simulink model "draftS_base"  (R2023b)
settings: Solver=ode4  StartTime=0.0  StopTime=0.5  FixedStep=Ts  RelTol=1e-3
undefined symbols (not defined in the file): Ts
libraries: spsMeanLib x7, spsCurrentMeasurementLib x4, spsVoltageMeasurementLib x3, spsSeriesRLCBranchLib x3, spsDCVoltageSourceLib x1, spsDiodeLib x1, spsGroundLib x1, spsMosfetLib x1, spsPWMGeneratorDCDCLib x1, sps_lib x1
settings Model: Creator=ssbor  LastModifiedBy=ssbor

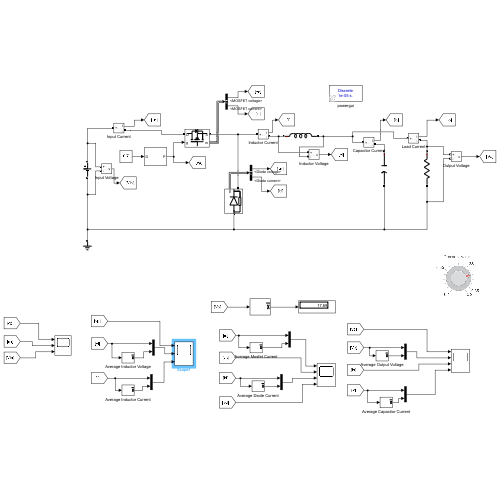
[thumbnail: Simulink's stored preview of the top-level diagram]
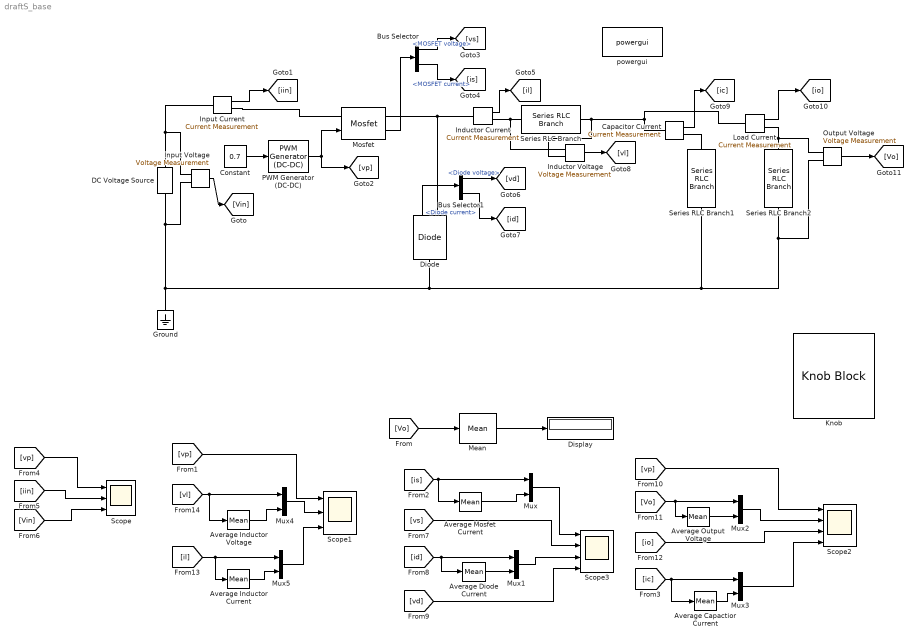
== system draftS_base ==
  Average Capactior Current : spsMeanLib/Mean  Freq=15000  Vinit=0  Ts=0
  Average Diode Current : spsMeanLib/Mean  Freq=15000  Vinit=0  Ts=0
  Average Inductor Current : spsMeanLib/Mean  Freq=15000  Vinit=0  Ts=0
  Average Inductor Voltage : spsMeanLib/Mean  Freq=15000  Vinit=0  Ts=0
      link override Model/Transport Delay: DelayTime=1./sps.Freq
  Average Mosfet Current : spsMeanLib/Mean  Freq=15000  Vinit=0  Ts=0
  Average Output Voltage : spsMeanLib/Mean  Freq=15000  Vinit=0  Ts=0
  Bus Selector : BusSelector  OutputSignals=MOSFET voltage,MOSFET current
  Bus Selector1 : BusSelector  OutputSignals=Diode voltage,Diode current
  Capacitor Current : spsCurrentMeasurementLib/Current Measurement  PhasorSimulation=off  OutputType=Complex  PSBequivalent=0
  Constant : Constant  Value=0.7
  DC Voltage Source : spsDCVoltageSourceLib/DC Voltage Source  Amplitude=25  Measurements=None
  Diode : spsDiodeLib/Diode  Ron=1e-7  Lon=0  Vf=0  IC=0  UseSnubber=0  Rs=1e6  Cs=1e6  Measurements=on
  Display : Display
  Ground : spsGroundLib/Ground  LConnTagsString=a
  Inductor Current : spsCurrentMeasurementLib/Current Measurement  PhasorSimulation=off  OutputType=Complex  PSBequivalent=0
  Inductor Voltage : spsVoltageMeasurementLib/Voltage Measurement  PhasorSimulation=off  OutputType=Complex  PSBequivalent=0
  Input Current : spsCurrentMeasurementLib/Current Measurement  PhasorSimulation=off  OutputType=Complex  PSBequivalent=0
  Input Voltage : spsVoltageMeasurementLib/Voltage Measurement  PhasorSimulation=off  OutputType=Complex  PSBequivalent=0
  Knob : KnobBlock  ScaleMin=0.1  ScaleMax=0.9  TickInterval=0.25
  Load Current : spsCurrentMeasurementLib/Current Measurement  PhasorSimulation=off  OutputType=Complex  PSBequivalent=0
  Mean : spsMeanLib/Mean  Freq=15000  Vinit=0  Ts=0
  Mosfet : spsMosfetLib/Mosfet  Ron=1e-7  Lon=0  Rd=1e-10  Vfd=0  IC=0  Rs=inf  Cs=0  Measurements=on
  Mux{,1..5} (6 alike) : Mux  Inputs=2
  Output Voltage : spsVoltageMeasurementLib/Voltage Measurement  PhasorSimulation=off  OutputType=Complex  PSBequivalent=0
  PWM Generator (DC-DC) : spsPWMGeneratorDCDCLib/PWM Generator (DC-DC)  Fsw=15000  Ts=Ts
  Scope : Scope  NumInputPorts=3
  Scope1 : Scope  NumInputPorts=3
  Scope2 : Scope  NumInputPorts=4
  Scope3 : Scope  NumInputPorts=4
  Series RLC Branch : spsSeriesRLCBranchLib/Series RLC Branch  LConnTagsString=__new0  RConnTagsString=__new0  BranchType=L  Resistance=1  Inductance=0.001  SetiL0=off  InitialCurrent=0  Capacitance=1e-6  Setx0=off  InitialVoltage=0  Measurements=None
  Series RLC Branch1 : spsSeriesRLCBranchLib/Series RLC Branch  LConnTagsString=__new0  RConnTagsString=__new0  BranchType=C  Resistance=1  Inductance=1e-3  SetiL0=off  InitialCurrent=0  Capacitance=470e-6  Setx0=off  InitialVoltage=0  Measurements=None
  Series RLC Branch2 : spsSeriesRLCBranchLib/Series RLC Branch  LConnTagsString=__new0  RConnTagsString=__new0  BranchType=R  Resistance=20  Inductance=1e-3  SetiL0=off  InitialCurrent=0  Capacitance=1e-6  Setx0=off  InitialVoltage=0  Measurements=None
  powergui : sps_lib/powergui  Priority=1  SimulationMode=Discrete  SampleTime=Ts  frequency=60  Iterations=50  frequencyindice=0  Pbase=100e6  ErrMax=1e-4  UnitsV=kV  UnitsW=MW  buscounter=0  FunctionMessages=off  echomessages=off  EnableUseOfTLC=off  CurrentSourceSwitches=off  DisableSnubberDevices=off  DisableRonSwitches=off  DisableVfSwitches=off  DisplayEquations=off  AutomaticDiscreteSolvers=off  SolverType=Tustin/Backward Euler (TBE)  Interpol=off  ExternalGateDelay=off  methode=off  Ts=100  x0status=blocks  SPID=on  SwTol=0  HookPort=off  NonlinearTolerance=1e-4  nMaxIteration=100  ContinueOnMaxIteration=off  RestoreLinks=warning  ResistiveCurrentMeasurement=off  Frange=[0:2:500]  Ylog=off  Xlog=on  ShowGrid=off  save=off  variable=ZData  structure=0  ZoomFFT=off  StartTime=0.0  cycles=1  DisplayStyle=1  fundamental=60  FreqAxis=off  MaxFrequency=1000  frequencyindicesteady=1  RmsSteady=1  display=off
  wires:
  Input Voltage/1 -> [Vin]
  Input Current/1 -> [iin]
  Constant/1 -> PWM Generator (DC-DC)/1
  PWM Generator (DC-DC)/1 -> [vp], Mosfet/1
  Mosfet/1 -> Bus Selector/1
  Bus Selector/1 -> [vs]  "<MOSFET voltage>"
  Bus Selector/2 -> [is]  "<MOSFET current>"
  Inductor Current/1 -> [il]
  Capacitor Current/1 -> [ic]
  Inductor Voltage/1 -> [vl]
  Load Current/1 -> [io]
  Output Voltage/1 -> [Vo]
  Diode/1 -> Bus Selector1/1
  Bus Selector1/1 -> [vd]  "<Diode voltage>"
  Bus Selector1/2 -> [id]  "<Diode current>"
  [Vo] -> Mean/1
  Mean/1 -> Display/1
  [vp] -> Scope/1
  [iin] -> Scope/2
  [Vin] -> Scope/3
  [vs] -> Scope3/2
  [vd] -> Scope3/4
  [vp] -> Scope2/1
  [io] -> Scope2/3
  Average Mosfet Current/1 -> Mux/2
  [is] -> Mux/1, Average Mosfet Current/1
  Mux/1 -> Scope3/1
  [id] -> Average Diode Current/1, Mux1/1
  Average Diode Current/1 -> Mux1/2
  Mux1/1 -> Scope3/3
  [Vo] -> Average Output Voltage/1, Mux2/1
  Average Output Voltage/1 -> Mux2/2
  Mux2/1 -> Scope2/2
  [ic] -> Average Capactior Current/1, Mux3/1
  Average Capactior Current/1 -> Mux3/2
  Mux3/1 -> Scope2/4
  [vp] -> Scope1/1
  [vl] -> Average Inductor Voltage/1, Mux4/1
  Average Inductor Voltage/1 -> Mux4/2
  Mux4/1 -> Scope1/2
  [il] -> Mux5/1, Average Inductor Current/1
  Average Inductor Current/1 -> Mux5/2
  Mux5/1 -> Scope1/3
  connections:
  DC Voltage Source/RConn1 -- Input Voltage/LConn1 -- Input Current/LConn1
  DC Voltage Source/LConn1 -- Input Voltage/LConn2 -- Ground/LConn1 -- Series RLC Branch2/RConn1 -- Output Voltage/LConn2 -- Series RLC Branch1/RConn1 -- Diode/LConn1
  Input Current/RConn1 -- Mosfet/LConn1
  Mosfet/RConn1 -- Diode/RConn1 -- Inductor Current/LConn1
  Inductor Current/RConn1 -- Inductor Voltage/LConn1 -- Series RLC Branch/LConn1
  Series RLC Branch/RConn1 -- Inductor Voltage/LConn2 -- Capacitor Current/LConn1 -- Load Current/LConn1
  Capacitor Current/RConn1 -- Series RLC Branch1/LConn1
  Load Current/RConn1 -- Output Voltage/LConn1 -- Series RLC Branch2/LConn1
